simulink model "test_RT"  (R2023a)
settings: Solver=FixedStepAuto  StartTime=0.0  StopTime=10.0  FixedStep=1  RelTol=1e-3
PreLoadFcn:
  | xt = importrobot('urdf\XT_PRU_noHands.urdf');
  | xt.DataFormat = 'col';
  | 
  | urdfPath = "urdf/XT_PRU_noHands.urdf";
libraries: robotmaniplib x3, RoboticsCode x2
settings Model: Creator=kgross  LastModifiedBy=speedgoat
settings SolverCC: ConcurrentTasks=on  PositivePriorityOrder=on
settings OptimizationCC: BlockReduction=off  OptimizeBlockIOStorage=off
settings DebuggingCC: TasksWithSamePriorityMsg=none
settings HardwareCC: ProdBitPerLong=64  ProdLongLongMode=on  ProdHWDeviceType=Intel->x86-64 (Linux 64)
settings SFSimCC: SimTargetLang=C++
settings RTWCC: Description=Simulink Real-Time  SystemTargetFile=slrealtime.tlc  TemplateMakefile=slrealtime_default_tmf  Toolchain=Simulink Real-Time Toolchain  BuildConfiguration=Faster Runs  CodeExecutionProfiling=on  TargetLang=C++

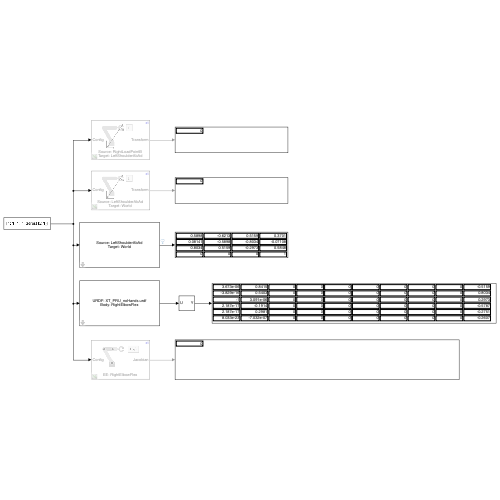
[thumbnail: Simulink's stored preview of the top-level diagram]
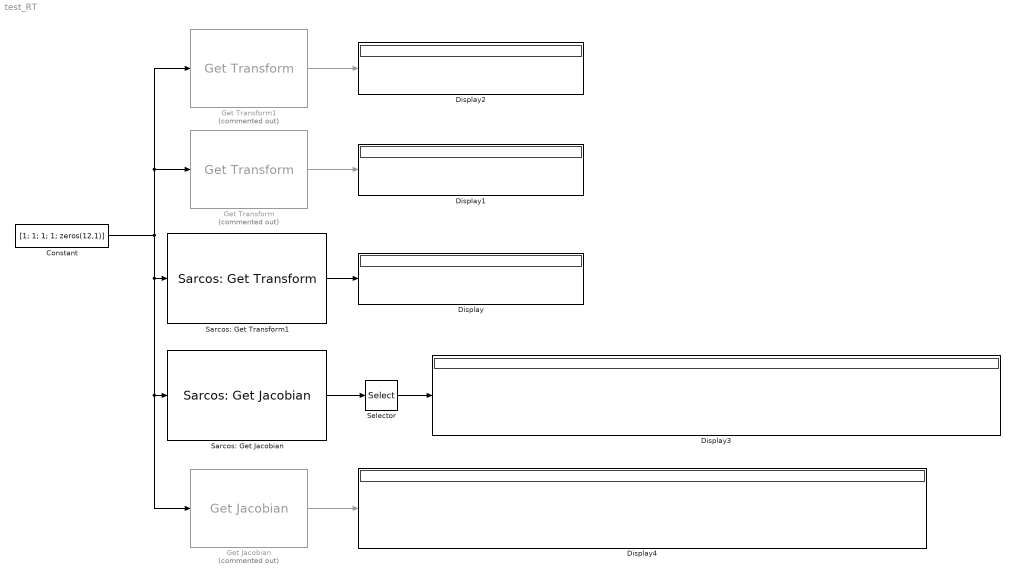
== system test_RT ==
  Constant : Constant  Value=[1; 1; 1; 1; zeros(12,1)]
  Display{,1..4} (5 alike) : Display
  Get Jacobian : robotmaniplib/Get Jacobian  Commented=on  RigidBodyTree=xt  EndEffector=RightElbowFlex  SimulateUsing=Interpreted execution
  Get Transform : robotmaniplib/Get Transform  Commented=on  RigidBodyTree=xt  SourceBody=LeftShoulderAbAd  TargetBody=World  SimulateUsing=Interpreted execution
  Get Transform1 : robotmaniplib/Get Transform  Commented=on  RigidBodyTree=xt  SourceBody=RightLoadPointB  TargetBody=LeftShoulderAbAd  SimulateUsing=Interpreted execution
  Sarcos: Get Jacobian : RoboticsCode/Sarcos: Get Jacobian  urdfpath='XT_PRU_noHands.urdf'  source=RightElbowFlex  source_string='RightElbowFlex'
  Sarcos: Get Transform1 : RoboticsCode/Sarcos: Get Transform  urdfpath='XT_PRU_noHands.urdf'  source=LeftShoulderAbAd  source_string='LeftShoulderAbAd'  target=World  target_string='World'
  Selector : Selector  NumberOfDimensions=2  InputPortWidth=3  IndexOptions=Select all,Index vector (dialog)  Indices=[1 3],1:16  OutputSizes=1,1
  wires:
  Constant/1 -> Sarcos: Get Transform1/1, Sarcos: Get Jacobian/1, Get Jacobian/1, Get Transform1/1, Get Transform/1
  Get Transform1/1 -> Display2/1
  Sarcos: Get Transform1/1 -> Display/1
  Get Jacobian/1 -> Display4/1
  Get Transform/1 -> Display1/1
  Selector/1 -> Display3/1
  Sarcos: Get Jacobian/1 -> Selector/1
